simulink model "roombaWheelExample"  (R2017b)
settings: Solver=VariableStepAuto  StartTime=0.0  StopTime=10.0  RelTol=1e-3
libraries: roombaCtrl x1
settings Model: Creator=wafflefries  LastModifiedBy=wafflefries

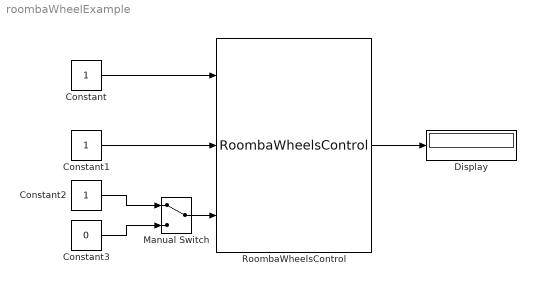
== system roombaWheelExample ==
  Constant : Constant
  Constant1 : Constant
  Constant2 : Constant
  Constant3 : Constant  Value=0
  Display : Display
  Manual Switch : ManualSwitch
  RoombaWheelsControl : roombaCtrl/RoombaWheelsControl
  wires:
  Manual Switch/1 -> RoombaWheelsControl/3
  Constant3/1 -> Manual Switch/2
  Constant2/1 -> Manual Switch/1
  Constant1/1 -> RoombaWheelsControl/2
  Constant/1 -> RoombaWheelsControl/1
  RoombaWheelsControl/1 -> Display/1
